simulink model "lqr_ex1_sim"  (R2023a)
settings: Solver=VariableStepAuto  StartTime=0.0  StopTime=20  RelTol=1e-3
values from neighbouring files (symbols this model uses):
  Ad = sysd_plant.A    [lqr_ex1.m]
  Bd = sysd_plant.B    [lqr_ex1.m]
  Cd = sysd_plant.C    [lqr_ex1.m]
  Dd = sysd_plant.D    [lqr_ex1.m]
  Nx = [1; 0]    [lqr_ex1.m]
  ref = 10    [lqr_ex1.m]
  Ts = 0.25    [lqr_ex1.m]
undefined symbols (not defined in the file or in its folder): Kgain
settings Model: Creator=Admin  LastModifiedBy=Admin
settings ModelReferenceCC: EnableRefExpFcnMdlSchedulingChecks=on

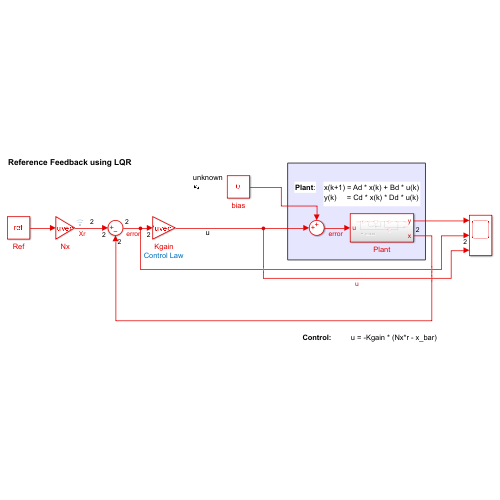
[thumbnail: Simulink's stored preview of the top-level diagram]
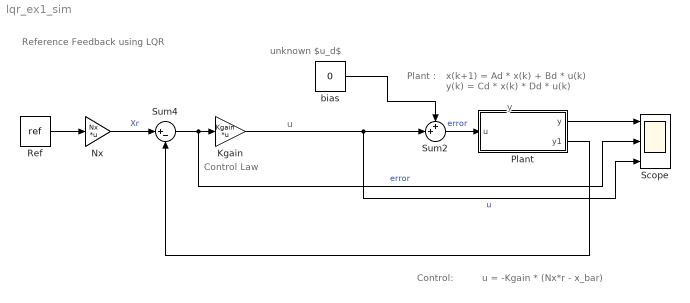
== system lqr_ex1_sim ==
  note: x(k+1) = Ad * x(k) + Bd * u(k)
      | y(k)     = Cd * x(k) * Dd * u(k)
  note: Plant :
  note: u = -Kgain * (Nx*r - x_bar)
  note: Control Law
  note: Reference Feedback using LQR
  note: unknown
      | $u_d$
  note: y
  note: u
  note: Control:
  Kgain : Gain  Gain=Kgain  Multiplication=Matrix(K*u) (u vector)
  Nx : Gain  Gain=Nx  Multiplication=Matrix(K*u) (u vector)
  Plant : Subsystem
  Ref : Constant  Value=ref  SampleTime=Ts
  Scope : Scope  NumInputPorts=3
  Sum2 : Sum  Inputs=++|
  Sum4 : Sum  Inputs=|+-
  bias : Constant  Value=0  SampleTime=Ts
  wires:
  Nx/1 -> Sum4/1  "Xr"
  Ref/1 -> Nx/1
  Sum4/1 -> Scope/2, Kgain/1  "error"
  Plant/1(y) -> Scope/1
  Sum2/1 -> Plant/1(u)  "error"
  Kgain/1 -> Scope/3, Sum2/2  "u"
  bias/1 -> Sum2/1
  Plant/2(y1) -> Sum4/2

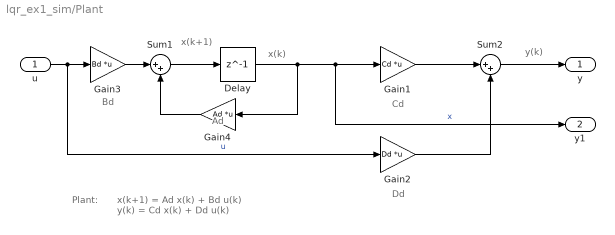
== system lqr_ex1_sim/Plant ==
  note: Plant:
  note: Dd
  note: x(k)
  note: x(k+1) = Ad x(k) + Bd u(k)
      | y(k) = Cd x(k) + Dd u(k)
  note: x(k+1)
  note: y(k)
  note: Ad
  note: Bd
  note: Cd
  u : Inport
  Delay : Delay  DelayLength=1
  Gain1 : Gain  Gain=Cd  Multiplication=Matrix(K*u) (u vector)
  Gain2 : Gain  Gain=Dd  Multiplication=Matrix(K*u) (u vector)
  Gain3 : Gain  Gain=Bd  Multiplication=Matrix(K*u) (u vector)
  Gain4 : Gain  Gain=Ad  Multiplication=Matrix(K*u) (u vector)
  Sum1 : Sum  Inputs=|++
  Sum2 : Sum  Inputs=|++
  y : Outport
  y1 : Outport  Port=2
  wires:
  u/1 -> Gain2/1, Gain3/1  "u"
  Sum1/1 -> Delay/1
  Delay/1 -> Gain4/1, y1/1, Gain1/1  "x"
  Gain3/1 -> Sum1/1
  Gain4/1 -> Sum1/2
  Sum2/1 -> y/1
  Gain1/1 -> Sum2/1
  Gain2/1 -> Sum2/2
